simulink model "ramp_response_simulink"  (R2019a)
settings: Solver=VariableStepAuto  StartTime=0.0  StopTime=45.0  RelTol=1e-3
libraries: simulink x1
settings Model: Creator=raxit  LastModifiedBy=raxit

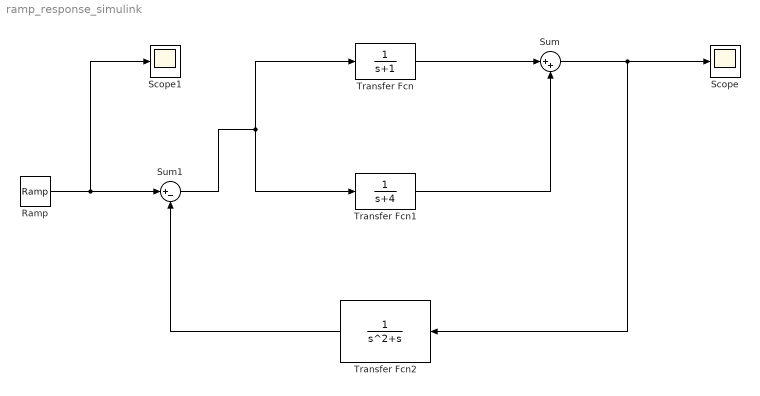
== system ramp_response_simulink ==
  Ramp : simulink/Sources/Ramp  slope=1  start=0  InitialOutput=0
  Scope : Scope
  Scope1 : Scope
  Sum : Sum  Inputs=|++
  Sum1 : Sum  Inputs=|+-
  Transfer Fcn : TransferFcn  Denominator=[1 1]
  Transfer Fcn1 : TransferFcn  Denominator=[1 4]
  Transfer Fcn2 : TransferFcn  Denominator=[1 1 0]
  wires:
  Ramp/1 -> Scope1/1, Sum1/1
  Transfer Fcn2/1 -> Sum1/2
  Sum1/1 -> Transfer Fcn1/1, Transfer Fcn/1
  Transfer Fcn/1 -> Sum/1
  Transfer Fcn1/1 -> Sum/2
  Sum/1 -> Transfer Fcn2/1, Scope/1
